simulink model "gmStateSpaceHDL_buckboost_convert_fixpt_vnl"  (R2025a)
settings: Solver=FixedStepDiscrete  StartTime=0.0  StopTime=0.005  FixedStep=Auto  RelTol=1e-3  AbsTol=1e-3
InitFcn:
  | load('C:\Users\bensa\Desktop\PI3_FPGA_BuckConverter\sschdl\buckboost_convert\stateSpaceParameters.mat');
values from neighbouring files (symbols this model uses):
  stateSpaceParameters_1 =     [stateSpaceParameters.mat]
libraries: fl_lib x5, hdlssclib x4, ee_lib x4, nesl_utility x4, simulink x3, hdlsllib x3
CloseFcn:
  | clear stateSpaceParameters_1
settings Model: MinMaxOverflowLogging=MinMaxAndOverflow  FPTRunName=EmbeddedRun1  Creator=bensa  LastModifiedBy=bensa
settings SolverCC: AutoScaleAbsTol=off  AlgebraicLoopSolver=TrustRegion  MaxZcPerStep=1.0
settings OptimizationCC: BlockReduction=off  ConditionallyExecuteInputs=off  DefaultParameterBehavior=Inlined  InheritOutputTypeSmallerThanSingle=on
settings DebuggingCC: SignalRangeChecking=warning  ArtificialAlgebraicLoopMsg=error  SingleTaskRateTransMsg=error  ParameterOverflowMsg=warning  ParameterUnderflowMsg=warning  UnconnectedInputMsg=warning  UnconnectedOutputMsg=warning  UnconnectedLineMsg=warning  SymbolicDimsDataTypeCodeGenerationDiagnostic=none
settings HardwareCC: ProdBitPerPointer=32.0  ProdBitPerSizeT=32.0  ProdBitPerPtrDiffT=32.0  ProdLargestAtomicFloat=None  ProdIntDivRoundTo=Undefined  ProdEndianess=Unspecified  ProdWordSize=32.0  ProdHWDeviceType=ASIC/FPGA->ASIC/FPGA  TargetBitPerPointer=64.0  TargetBitPerSizeT=64.0  TargetBitPerPtrDiffT=64.0  TargetLongLongMode=on  TargetIntDivRoundTo=Zero  TargetEndianess=LittleEndian  TargetWordSize=64.0  TargetHWDeviceType=Custom Processor->MATLAB Host Computer  ProdEqTarget=off
settings ModelReferenceCC: EnableRefExpFcnMdlSchedulingChecks=on
settings SFSimCC: CustomCodeUndefinedFunction=UseInterfaceOnly
settings RTWCC: GPUComputeCapability=3.5  DLArmComputeVersion=19.05
settings SimscapeCC: SimscapeLogType=all  SimscapeLogSimulationStatistics=on  SimscapeLogDataHistory=10000.0

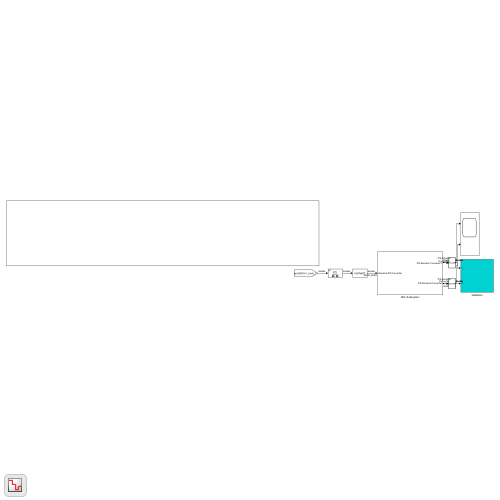
[thumbnail: Simulink's stored preview of the top-level diagram]
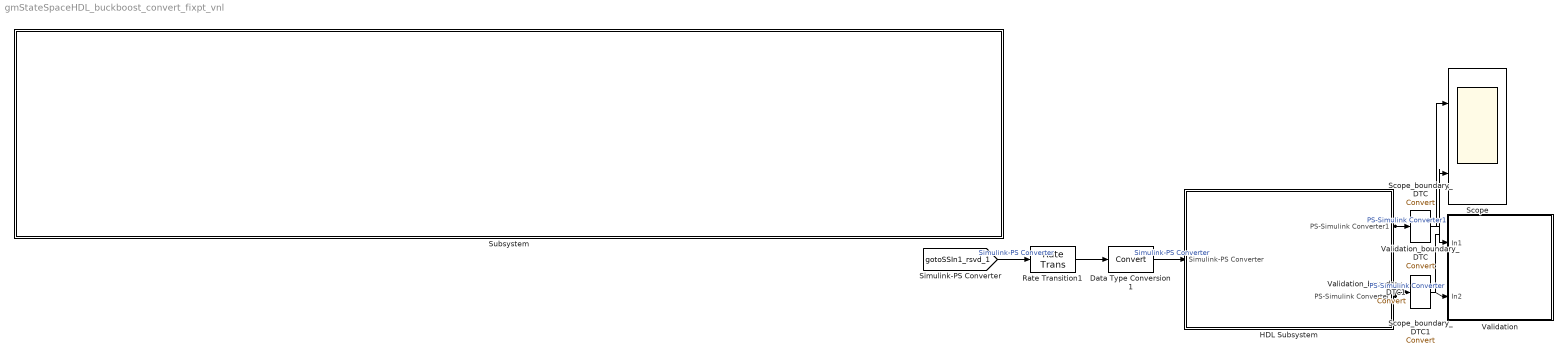
== system gmStateSpaceHDL_buckboost_convert_fixpt_vnl ==
  Data Type Conversion1 : DataTypeConversion  RndMeth=Nearest  SaturateOnIntegerOverflow=off
  HDL Subsystem : Subsystem  DataTypeOverride=Off  MinMaxOverflowLogging=MinMaxAndOverflow
  Rate Transition1 : RateTransition  OutPortSampleTime=5e-08
  Scope : Scope  NumInputPorts=2
      settings: DataLoggingVariableName=ScopeData2  DataLoggingSaveFormat=Array
  Scope_boundary_DTC : DataTypeConversion
  Scope_boundary_DTC1 : DataTypeConversion
  Subsystem : Subsystem
  Validation : Subsystem
  Validation_boundary_DTC : DataTypeConversion
  Validation_boundary_DTC1 : DataTypeConversion
  wires:
  HDL Subsystem/2(PS-Simulink Converter) -> Scope_boundary_DTC1/1, Validation_boundary_DTC1/1  "PS-Simulink Converter"
  Data Type Conversion1/1 -> HDL Subsystem/1(Simulink-PS Converter)  "Simulink-PS Converter"
  [gotoSSIn1_rsvd_1] -> Rate Transition1/1  "Simulink-PS Converter"
  Rate Transition1/1 -> Data Type Conversion1/1
  HDL Subsystem/1(PS-Simulink Converter1) -> Scope_boundary_DTC/1, Validation_boundary_DTC/1  "PS-Simulink Converter1"
  Scope_boundary_DTC/1 -> Scope/1
  Validation_boundary_DTC/1 -> Validation/1(In1)
  Scope_boundary_DTC1/1 -> Scope/2
  Validation_boundary_DTC1/1 -> Validation/2(In2)

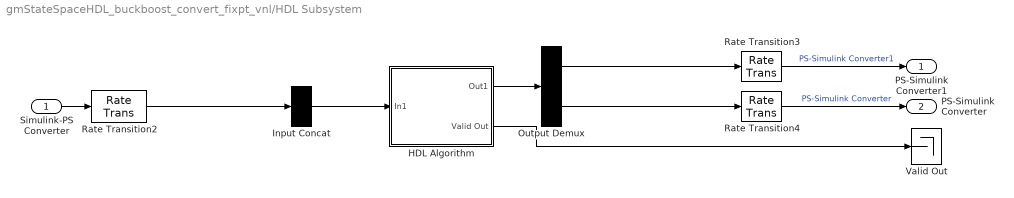
== system gmStateSpaceHDL_buckboost_convert_fixpt_vnl/HDL Subsystem ==
  Simulink-PS Converter : Inport  OutDataTypeStr=fixdt(0,32,29)
  HDL Algorithm : Subsystem
  Input Concat : Concatenate  NumInputs=1
  Output Demux : Demux  Outputs=2
  Rate Transition2 : RateTransition  Integrity=off  OutPortSampleTimeOpt=Multiple of input port sample time  OutPortSampleTimeMultiple=1/2
  Rate Transition3 : RateTransition  OutPortSampleTimeOpt=Multiple of input port sample time  OutPortSampleTimeMultiple=2
  Rate Transition4 : RateTransition  OutPortSampleTimeOpt=Multiple of input port sample time  OutPortSampleTimeMultiple=2
  Valid Out : Terminator
  PS-Simulink Converter1 : Outport
  PS-Simulink Converter : Outport  Port=2
  wires:
  Rate Transition3/1 -> PS-Simulink Converter1/1  "PS-Simulink Converter1"
  HDL Algorithm/1(Out1) -> Output Demux/1
  Input Concat/1 -> HDL Algorithm/1(In1)
  HDL Algorithm/2(Valid Out) -> Valid Out/1
  Rate Transition2/1 -> Input Concat/1
  Simulink-PS Converter/1 -> Rate Transition2/1
  Output Demux/2 -> Rate Transition4/1
  Output Demux/1 -> Rate Transition3/1
  Rate Transition4/1 -> PS-Simulink Converter/1  "PS-Simulink Converter"

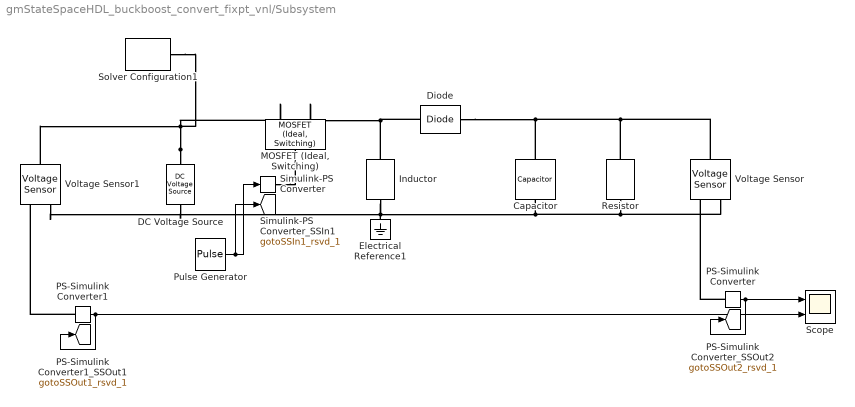
== system gmStateSpaceHDL_buckboost_convert_fixpt_vnl/Subsystem ==
  Capacitor : fl_lib/Electrical/Electrical Elements/Capacitor  c=47 uF  r=1e-6 Ohm  g=0 1/Ohm  i_specify=off  i_priority=None  i=0 A  i_nominal_specify=off  i_nominal_value=1  i_nominal_unit=A  v_specify=off  v_priority=None  v=0 V  v_nominal_specify=off  v_nominal_value=1  v_nominal_unit=V  vc_specify=off  vc_priority=High  vc=0 V  vc_nominal_specify=off  vc_nominal_value=1  vc_nominal_unit=V
  DC Voltage Source : ee_lib/Additional Components/SPICE Sources/DC Voltage Source  DC=5 V
  Diode : ee_lib/Semiconductors & Converters/Diode  ModelType=ee.enum.diode.modelType.pwl  TableType=ee.enum.diode.tableType.IfMat  IfMat=[.07, .12, .19, 1.75, 4.24, 7.32, 11.2; .16, .3, .72, 2.14, 5.02, 8.35, 13.12] A  VfMat=[.9, 1.15, 1.25, 1.5, 1.75, 2.17, 2.6, 2.85; .58, .68, .75, 1.1, 1.38, 1.77, 2.27, 2.7] V  TjVec=[25, 125] degC  VfVec=[.5, .7, .9, 1.3, 1.7, 2.1, 2.5] V  IfVec=[.1, .2, .5, 1, 2, 4, 7, 10] A  IrMat=[1e-06, 2e-06, 5e-06, 1e-05, 2.5e-05, 5e-05, .0001; 2e-06, 5e-06, 1e-05, 4e-05, 8e-05, .0002, .0005] A  VrMat=[10, 100, 200, 250, 300, 325, 350; 10, 70, 160, 220, 270, 300, 320] V  VrVec=[10, 20, 40, 50, 70, 80, 100] V  IrVec=[1e-06, 2e-06, 5e-06, 1e-05, 2e-05, 5e-05, .0001] A  Vf=0.7 V  Ron=0.1 Ohm  Goff=1e-8 S  prmExp=ee.enum.diode.expParam.useTwo  I12=[.0137, .545] A  V12=[.6, .7] V  RS=0 Ohm  Tmeas=298.15 K  IS=1e-12 A  ec=1  I1=0.0137 A  V1=0.6 V  N_series=1  N_parallel=1  ZenerEnable=false  Rz=0.3 Ohm  BV=inf V  C_param=ee.enum.diode.capParam.fixed  CJ=0 pF  CJ0=5 pF  Vvec=[.1, 10, 100] V  Cvec=[3.5, 1, .4] pF  VJ=1 V  Mgrad=0.5  FC=0.5  Q_param=ee.enum.diode.recoveryParam.off  iRM=-7.15 A  iF=4 A  didt=-750 A/us  trr_factor=3  trr=115 ns  Qrr=150 nA*s  Vr=-600 V  Ls=150 nH  Erec=0.03 J  TT=50 ns  tau=100 ns  T_param=ee.enum.diode.temperatureParam.off  Tdevice=298.15 K  I1_T2=0.245 A  V1_T2=0.5 V  IS_T2=1.25e-7 A  Tmeas2=125 degC  XTI_param=ee.enum.diode.xtiParam.pn  XTI=3  EG_param=ee.enum.diode.egapParam.material_si  EG=1.11 eV  dBVdT=0 V/K  enable_fault_input=simscape.enum.onoff.off  i_specify=off  i_priority=None  i=0 A  i_nominal_specify=off  i_nominal_value=1  i_nominal_unit=A  v_specify=off  v_priority=None  v=0 V  v_nominal_specify=off  v_nominal_value=1  v_nominal_unit=V  v_capacitor_specify=off  v_capacitor_priority=None  v_capacitor=0 V  v_capacitor_nominal_specify=off  v_capacitor_nominal_value=1  v_capacitor_nominal_unit=V  Qj_specify=off  Qj_priority=High  Qj=0 C  Qj_nominal_specify=off  Qj_nominal_value=1  Qj_nominal_unit=C  i_diode_specify=off  i_diode_priority=None  i_diode=0 A  i_diode_nominal_specify=off  i_diode_nominal_value=1  i_diode_nominal_unit=A  v_diode_specify=off  v_diode_priority=None  v_diode=0 V  v_diode_nominal_specify=off  v_diode_nominal_value=1  v_diode_nominal_unit=V  i_capacitor_specify=off  i_capacitor_priority=None  i_capacitor=0 A  i_capacitor_nominal_specify=off  i_capacitor_nominal_value=1  i_capacitor_nominal_unit=A  power_dissipated_specify=off  power_dissipated_priority=None  power_dissipated=0 W  power_dissipated_nominal_specify=off  power_dissipated_nominal_value=1  power_dissipated_nominal_unit=W  fidelity_level=ee.enum.diode.fidelity.includeChargeDyn  rec_loss_model=ee.enum.diode.reverseRecoveryModel.fixed  ErecVal=0 J  scaleWithIandV=true  ErecMat=zeros(2, 3) J  TjrecVec=[298.15, 398.15] K  IfrecVec=[.1, 1, 10] A  IrecVal=10 A  VrecVal=10 V  tFilter=1 / 1000 / 100 s  thermal_network_parameterization=ee.enum.thermalNetworkTopology.junctionCase  Rth=[0, 10] K/W  Rth_Cauer=[1, 3, 10] K/W  Rth_Foster=[.08, .14, .22, .16] K/W  thermal_mass_parameterization=ee.enum.thermalNetwork.timeconstant  thermal_mass=[0, 1] J/K  thermal_mass_Cauer=[.1, .3, 1] J/K  thermal_mass_Foster=[.001, .005, .05, .5] J/K  thermal_time_constant=[0, 10] s  thermal_time_constant_Cauer=[1, 3, 10] s  thermal_time_constant_Foster=[7e-05, .0007, .01, .08] s  thermal_mass_initial_temperatures=[25, 25] degC  thermal_mass_initial_temperatures_Cauer=[25, 25, 25] degC  junction_thermal_mass=0.01 J/K  Tvec_initial_Foster=[25, 25, 25, 25] degC  no_thermal_network=0  junction_temperature_specify=off  junction_temperature_priority=None  junction_temperature=25 degC  junction_temperature_nominal_specify=off  junction_temperature_nominal_value=1  junction_temperature_nominal_unit=degC
  Electrical Reference1 : fl_lib/Electrical/Electrical Elements/Electrical Reference
  Inductor : ee_lib/Passive/Inductor  l=100 uH  enable_L_tol=ee.enum.toleranceApplication.none  L_tol=20  tol_distribution=ee.enum.toleranceDistribution.uniform  nSigma=4  r=0 Ohm  g=1e-9 1/Ohm  enable_operating_limits=ee.enum.enable.no  operating_limit_action=ee.enum.passive.reportOpLim.warn  max_working_current=1 A  power_rating=1 W  i_L_specify=off  i_L_priority=High  i_L=0 A  i_L_nominal_specify=off  i_L_nominal_value=1  i_L_nominal_unit=A
  "MOSFET (Ideal, Switching)" : ee_lib/Semiconductors & Converters/MOSFET (Ideal, Switching)  port_option=ee.enum.controlport.ps  Rds=0.01 Ohm  Goff=1e-6 1/Ohm  Vth=2 V  diode_param=ee.enum.semiconductors.protectionDiode.external  diode_Vf=0.8 V  diode_Ron=0.001 Ohm  diode_Goff=1e-5 1/Ohm  diode_C=50e-9 F  diode_iRM=-235 A  diode_iF=300 A  diode_idot=-50 A/us  diode_trr_param=ee.enum.converters.diodeReverseParam.trr_factor  diode_trr_factor=3  diode_trr=15 us  diode_Qrr=1500 s*uA  ids_specify=off  ids_priority=None  ids=0 A  ids_nominal_specify=off  ids_nominal_value=1  ids_nominal_unit=A  vds_specify=off  vds_priority=None  vds=0 V  vds_nominal_specify=off  vds_nominal_value=1  vds_nominal_unit=V  vgs_specify=off  vgs_priority=None  vgs=0 V  vgs_nominal_specify=off  vgs_nominal_value=1  vgs_nominal_unit=V  thermal_loss_option=ee.enum.converters.thermalLossOption.constantvalues  Von_data=[0, 1.8, 3.2, 6, 10, 16; 0, 2, 5.5, 9.5, 15, 25] V  Tj=[298.15, 448.15] K  Iout_data=[0, 20, 40, 60, 80, 100] A  Eon_data=[0, 55.04, 124.57, 235.53, 362.12; 0, 71.25, 161.25, 304.88, 468.75] * 1e-6 J  Eoff_data=[0, 18, 30, 56.1, 76.5; 0, 22.5, 37.5, 70.13, 95.63] * 1e-6 J  Eon_data_3D=[zeros(2, 5, 3)] J  Eoff_data_3D=[zeros(2, 5, 3)] J  Tj_loss=[298.15, 448.15] K  Iout_data_loss=[0, 10, 20, 30, 40] A  tabulateWithVds=false  Vds_loss=[0, 150, 300] V  Eon_scalar=22.86e-3 J  Eoff_scalar=17.14e-3 J  Voff=300 V  Iout_scalar=600 A  useCurrentFromPreviousCycle=false  useVoltageFromPreviousCycle=false  diodeModelType=ee.enum.converters.diodeModelType.pwl  diodeTableType=ee.enum.diode.tableType.IfMat  diode_ReverseIVType=ee.enum.diode.diodeReverseIV.constant  diode_IfMat=[.07, .12, .19, 1.75, 4.24, 7.32, 11.2; .16, .3, .72, 2.14, 4.02, 6.35, 9.12] A  diode_VfMat=[.9, 1.15, 1.25, 1.5, 1.75, 2.17, 2.6, 2.85; .58, .68, .75, 1.1, 1.38, 1.77, 2.27, 2.7] V  diode_TjVec=[25, 125] degC  diode_VfVec=[.5, .7, .9, 1.3, 1.7, 2.1, 2.5] V  diode_IfVec=[.1, .2, .5, 1, 2, 4, 7, 10] A  diode_IrMat=[1e-06, 2e-06, 5e-06, 1e-05, 2.5e-05, 5e-05, .0001; 2e-06, 5e-06, 1e-05, 4e-05, 8e-05, .0002, .0005] A  diode_VrMat=[10, 100, 200, 250, 300, 325, 350; 10, 70, 160, 220, 270, 300, 320] V  diode_VrVec=[10, 20, 40, 50, 70, 80, 100] V  diode_IrVec=[1e-06, 2e-06, 5e-06, 1e-05, 2e-05, 5e-05, .0001] A  diode_Vr=-600 V  diode_Ls=150 nH  diode_Erec=0.03 J  diode_rec_loss_model=ee.enum.diode.reverseRecoveryModel.fixed  diode_ErecVal=0 J  diode_scaleWithIandV=true  diode_ErecMat=zeros(2, 3) J  diode_TjrecVec=[298.15, 398.15] K  diode_IfrecVec=[.1, 1, 10] A  diode_IrecVal=10 A  diode_VrecVal=10 V  diode_tFilter=1 / 1000 / 100 s  separateThermalPortForDiode=false  thermal_network_parameterization=ee.enum.thermalNetworkTopology.external  Rth=[.03, .2] K/W  Rth_Cauer=[.03, .1, .2] K/W  Rth_Foster=[.08, .14, .22, .16] K/W  thermal_mass_parameterization=ee.enum.thermalNetwork.timeconstant  thermal_mass=[3, 25] J/K  thermal_mass_Cauer=[3, 10, 25] J/K  thermal_mass_Foster=[.001, .005, .05, .5] J/K  thermal_time_constant=[.1, 5] s  thermal_time_constant_Cauer=[.1, 1, 5] s  thermal_time_constant_Foster=[7e-05, .0007, .01, .08] s  thermal_mass_initial_temperatures=[25, 25] degC  thermal_mass_initial_temperatures_Cauer=[25, 25, 25] degC  junction_thermal_mass=0.1 J/K  Tvec_initial_Foster=[25, 25, 25, 25] degC  RthDiode=[.03, .2] K/W  RthCauerDiode=[.03, .1, .2] K/W  RthFosterDiode=[.03, .2] K/W  thermalMassDiode=[3, 25] J/K  thermalMassCauerDiode=[3, 10, 25] J/K  thermalMassFosterDiode=[33, 50] J/K  thermalTauDiode=[.1, 5] s  thermalTauCauerDiode=[.1, 1, 5] s  thermalTauFosterDiode=[1, 10] s  thermalMassInitTempDiode=[25, 25] degC  thermalMassInitTempCauerDiode=[25, 25, 25] degC  junctionthermalMassDiode=0.1 J/K  TVecInitialFosterDiode=[25, 25, 25, 25] degC  no_thermal_network=0  mosfet_junction_temperature_specify=off  mosfet_junction_temperature_priority=None  mosfet_junction_temperature=25 degC  mosfet_junction_temperature_nominal_specify=off  mosfet_junction_temperature_nominal_value=1  mosfet_junction_temperature_nominal_unit=degC  diode_junction_temperature_specify=off  diode_junction_temperature_priority=None  diode_junction_temperature=25 degC  diode_junction_temperature_nominal_specify=off  diode_junction_temperature_nominal_value=1  diode_junction_temperature_nominal_unit=degC  Qj_specify=off  Qj_priority=None  Qj=0 W  Qj_nominal_specify=off  Qj_nominal_value=1  Qj_nominal_unit=W  accumulatedSwitchingLosses_specify=off  accumulatedSwitchingLosses_priority=None  accumulatedSwitchingLosses=0 J
  PS-Simulink Converter : nesl_utility/PS-Simulink Converter  PhysicalDomain=network_engine_domain  SubClassName=ps_output  LeftPortType=input  RightPortType=output  PseudoPeriodic=off  Frequencies=[]  VectorFormat=inherit  Unit=inherit  AffineConversion=off
  PS-Simulink Converter1 : nesl_utility/PS-Simulink Converter  PhysicalDomain=network_engine_domain  SubClassName=ps_output  LeftPortType=input  RightPortType=output  PseudoPeriodic=off  Frequencies=[]  VectorFormat=inherit  Unit=inherit  AffineConversion=off
  Pulse Generator : DiscretePulseGenerator  Amplitude=5  Period=200  PulseWidth=.40*200  SampleTime=50e-9
  Resistor : fl_lib/Electrical/Electrical Elements/Resistor  R=24 Ohm  i_specify=off  i_priority=None  i=0 A  i_nominal_specify=off  i_nominal_value=1  i_nominal_unit=A  v_specify=off  v_priority=None  v=0 V  v_nominal_specify=off  v_nominal_value=1  v_nominal_unit=V
  Scope : Scope  NumInputPorts=2
      settings: ActiveDisplayYMinimum=-5.8064728350082557  ActiveDisplayYMaximum=6.2007192038898058
  Simulink-PS Converter : nesl_utility/Simulink-PS Converter  PhysicalDomain=network_engine_domain  SubClassName=ps_input  LeftPortType=input  RightPortType=output  PseudoPeriodic=off  Frequencies=[]  NoiseDistribution=none  NoiseParameters=[]  Unit=1  AffineConversion=off  FilteringAndDerivatives=provide  SimscapeFilterOrder=1  InputFilterTimeConstant=0.001  UdotUserProvided=0
  Solver Configuration1 : nesl_utility/Solver Configuration  PhysicalDomain=network_engine_domain  SubClassName=solver  LeftPortType=input  RightPortType=generic  Tones=[]  Harmonics=[]  SimulateNoise=off  Profile=off  UseLocalSampling=off  EnableSwitchedLinearOptims=on  FrequencyDomain=off  UseCCode=off  RelTol=0.001  AbsTol=0.001  MinStep=1e-09  ToWorkspace=off  RevertToSquareIcSolve=off  NumHomotopyIterations=100  PhasorMode=off  PhasorModeNumHarmonics=1  ConsistencySolver=NEWTON_XTOL_AFTER_FTOL  IndexReductionMethod=DerivativeReplacement  DoDC=off  ResidualTolerance=1e-09  ConsistencyTolSource=GLOBAL  ConsistencyAbsTol=0.001  ConsistencyRelTol=0.001  ConsistencyTolFactor=0.001  UseLocalSolver=on  LocalSolverChoice=NE_BACKWARD_EULER_ADVANCER  ResolveIndetEquations=on  FunctionEvalNumThread=1  LocalSolverSampleTime=50e-9  DoFixedCost=on  MaxNonlinIter=2  MaxModeIter=2  ComputeImpulses=off  ImpulseIterations=2  LinearAlgebra=auto  LinearAlgebraNumThread=0  EquationFormulation=NE_TIME_EF  DelaysMemoryBudget=1024  AutomaticFiltering=on  FilteringTimeConstant=0.001  PartitionStorageMethod=AS_NEEDED  PartitionMemoryBudget=1024  PartitionMethod=ROBUST  MultibodyUseLocalSolver=off  MultibodyLocalSolverChoice=ODE1  MultibodyLocalSolverSampleTime=0.001
  Voltage Sensor : fl_lib/Electrical/Electrical Sensors/Voltage Sensor
  Voltage Sensor1 : fl_lib/Electrical/Electrical Sensors/Voltage Sensor
  tag scope: gotoSSIn1_rsvd_1=global, gotoSSOut1_rsvd_1=global, gotoSSOut2_rsvd_1=global
  wires:
  Pulse Generator/1 -> Simulink-PS Converter/1, [gotoSSIn1_rsvd_1]
  PS-Simulink Converter1/1 -> Scope/2, [gotoSSOut1_rsvd_1]
  PS-Simulink Converter/1 -> Scope/1, [gotoSSOut2_rsvd_1]
  connections:
  Voltage Sensor/LConn1 -- Capacitor/LConn1 -- Diode/LConn1 -- Resistor/LConn1
  Voltage Sensor/RConn2 -- Capacitor/RConn1 -- Electrical Reference1/LConn1 -- Inductor/RConn1 -- Voltage Sensor1/RConn2 -- DC Voltage Source/RConn1 -- Resistor/RConn1
  PS-Simulink Converter/LConn1 -- Voltage Sensor/RConn1
  DC Voltage Source/LConn1 -- "MOSFET (Ideal, Switching)"/RConn1 -- Solver Configuration1/RConn1 -- Voltage Sensor1/LConn1
  PS-Simulink Converter1/LConn1 -- Voltage Sensor1/RConn1
  Inductor/LConn1 -- "MOSFET (Ideal, Switching)"/RConn2 -- Diode/RConn1
  Simulink-PS Converter/RConn1 -- "MOSFET (Ideal, Switching)"/LConn1

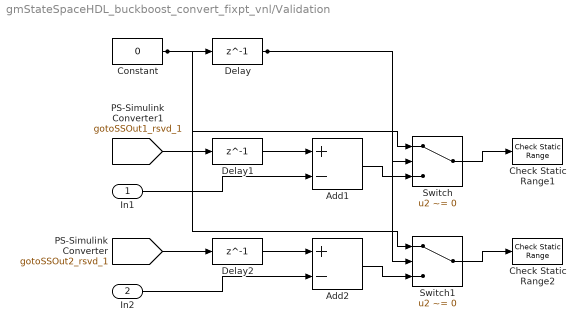
== system gmStateSpaceHDL_buckboost_convert_fixpt_vnl/Validation ==
  In1 : Inport
  In2 : Inport  Port=2
  Add1 : Sum  Inputs=+-
  Add2 : Sum  Inputs=+-
  Check Static Range1 : simulink/Model Verification/Check  Static Range  Description=-0.001 <= u <= 0.001  max=0.001  max_included=on  min=-0.001  min_included=on  enabled=on  stopWhenAssertionFail=off  export=off  icon=graphic
      settings: LibrarySourceBlock=|
      | hdlsllib/Model
      | Verification/Check
      | Static Range
  Check Static Range2 : simulink/Model Verification/Check  Static Range  Description=-0.001 <= u <= 0.001  max=0.001  max_included=on  min=-0.001  min_included=on  enabled=on  stopWhenAssertionFail=off  export=off  icon=graphic
      settings: LibrarySourceBlock=|
      | hdlsllib/Model
      | Verification/Check
      | Static Range
  Constant : Constant  Value=0  SampleTime=5e-08
  Delay : Delay  DelayLength=1  InitialCondition=1
  Delay1 : Delay  DelayLength=1
  Delay2 : Delay  DelayLength=1
  Switch : Switch  Criteria=u2 ~= 0  SaturateOnIntegerOverflow=off  InputSameDT=off
  Switch1 : Switch  Criteria=u2 ~= 0  SaturateOnIntegerOverflow=off  InputSameDT=off
  wires:
  Constant/1 -> Delay/1, Switch/1, Switch1/1
  [gotoSSOut1_rsvd_1] -> Delay1/1
  Delay1/1 -> Add1/1
  In1/1 -> Add1/2
  Add1/1 -> Switch/3
  Delay/1 -> Switch/2, Switch1/2
  Switch/1 -> Check Static Range1/1
  [gotoSSOut2_rsvd_1] -> Delay2/1
  Delay2/1 -> Add2/1
  In2/1 -> Add2/2
  Add2/1 -> Switch1/3
  Switch1/1 -> Check Static Range2/1

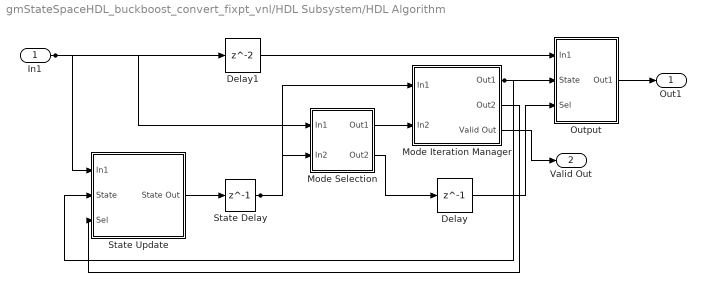
== system gmStateSpaceHDL_buckboost_convert_fixpt_vnl/HDL Subsystem/HDL Algorithm ==
  In1 : Inport  OutDataTypeStr=fixdt(0,32,29)
  Delay : Delay  DelayLength=1
  Delay1 : Delay
  Mode Iteration Manager : Subsystem
  Mode Selection : Subsystem
  Output : Subsystem
  State Delay : Delay  DelayLength=1  InitialCondition=single(stateSpaceParameters_1.X0)
  State Update : Subsystem
  Out1 : Outport  VectorParamsAs1DForOutWhenUnconnected=off
  Valid Out : Outport  Port=2  VectorParamsAs1DForOutWhenUnconnected=off
  wires:
  State Delay/1 -> Mode Iteration Manager/1(In1), Mode Selection/2(In2)
  Delay1/1 -> Output/1(In1)
  State Update/1(State Out) -> State Delay/1
  In1/1 -> Mode Selection/1(In1), Delay1/1, State Update/1(In1)
  Mode Selection/1(Out1) -> Mode Iteration Manager/2(In2)
  Mode Iteration Manager/2(Out2) -> State Update/3(Sel)
  Mode Iteration Manager/1(Out1) -> State Update/2(State), Output/2(State)
  Mode Selection/2(Out2) -> Delay/1
  Mode Iteration Manager/3(Valid Out) -> Valid Out/1
  Output/1(Out1) -> Out1/1
  Delay/1 -> Output/3(Sel)

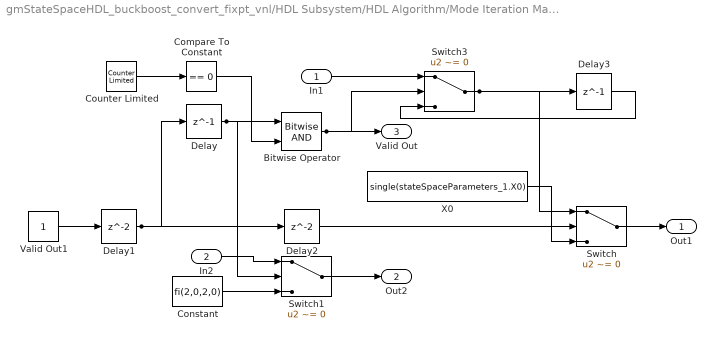
== system gmStateSpaceHDL_buckboost_convert_fixpt_vnl/HDL Subsystem/HDL Algorithm/Mode Iteration Manager ==
  In1 : Inport  LockScale=on
  In2 : Inport  Port=2  OutDataTypeStr=fixdt(0,2,0)  LockScale=on
  Bitwise Operator : simulink/Logic and Bit Operations/Bitwise Operator  logicop=AND  UseBitMask=off  NumInputPorts=2  BitMask=bin2dec('11011001')  BitMaskRealWorld=Stored Integer
      settings: LibrarySourceBlock=|
      | hdlsllib/Logic and Bit
      | Operations/Bitwise
      | Operator
  Compare To Constant : hdlsllib/Logic and Bit Operations/Compare To Constant  relop===  const=0  OutDataTypeStr=boolean
  Constant : Constant  Value=fi(2,0,2,0)  SampleTime=2.5e-08  LockScale=on
  Counter Limited : hdlsllib/Sources/Counter Limited  uplimit=1  tsamp=-1
  Delay : Delay  DelayLength=1
  Delay1 : Delay
  Delay2 : Delay
  Delay3 : Delay  DelayLength=1
  Switch : Switch  Criteria=u2 ~= 0  OutDataTypeStr=fixdt(1,32,25)  SaturateOnIntegerOverflow=off  InputSameDT=off
  Switch1 : Switch  Criteria=u2 ~= 0  SaturateOnIntegerOverflow=off  InputSameDT=off  OutDataTypeStr=Inherit: Same as first input
      settings: LockScale=on
  Switch3 : Switch  Criteria=u2 ~= 0  OutDataTypeStr=fixdt(1,32,28)  SaturateOnIntegerOverflow=off  InputSameDT=off
  Valid Out1 : Constant  OutDataTypeStr=boolean  SampleTime=2.5e-08
  X0 : Constant  Value=single(stateSpaceParameters_1.X0)  OutDataTypeStr=fixdt(0,32,29)  SampleTime=2.5e-08
  Out1 : Outport  OutDataTypeStr=fixdt(1,32,25)  VectorParamsAs1DForOutWhenUnconnected=off
  Out2 : Outport  Port=2  VectorParamsAs1DForOutWhenUnconnected=off
  Valid Out : Outport  Port=3  VectorParamsAs1DForOutWhenUnconnected=off
  wires:
  Valid Out1/1 -> Delay1/1
  Counter Limited/1 -> Compare To Constant/1
  Delay1/1 -> Delay/1, Delay2/1
  Compare To Constant/1 -> Bitwise Operator/2
  Delay/1 -> Switch1/2, Bitwise Operator/1
  In2/1 -> Switch1/1
  Constant/1 -> Switch1/3
  In1/1 -> Switch3/1
  Bitwise Operator/1 -> Valid Out/1, Switch3/2
  Delay2/1 -> Switch/2
  Switch1/1 -> Out2/1
  Switch3/1 -> Delay3/1, Switch/1
  X0/1 -> Switch/3
  Delay3/1 -> Switch3/3
  Switch/1 -> Out1/1

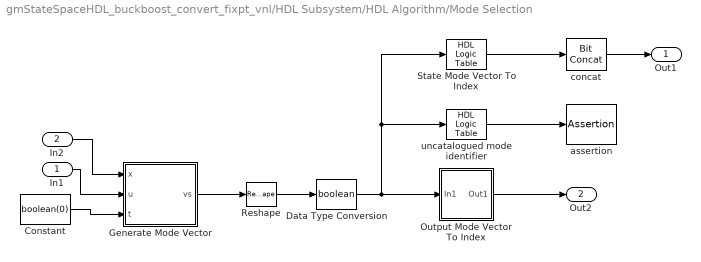
== system gmStateSpaceHDL_buckboost_convert_fixpt_vnl/HDL Subsystem/HDL Algorithm/Mode Selection ==
  In1 : Inport  OutDataTypeStr=fixdt(0,32,29)
  In2 : Inport  Port=2  LockScale=on
  Constant : Constant  Value=boolean(0)  SampleTime=2.5e-08
  Data Type Conversion : DataTypeConversion  OutDataTypeStr=boolean  RndMeth=Nearest  SaturateOnIntegerOverflow=off
  Generate Mode Vector : Subsystem  TreatAsAtomicUnit=on  Variant=on
  Output Mode Vector To Index : Subsystem
  Reshape : Reshape
  State Mode Vector To Index : hdlssclib/HDL Logic Table  InputTable=stateSpaceParameters_1.logicTableInput  OutputTable=stateSpaceParameters_1.logicTableOutput
  assertion : Assertion  StopWhenAssertionFail=off
  concat : hdlsllib/Logic and Bit Operations/Bit Concat  numInputs=1
  uncatalogued mode identifier : hdlssclib/HDL Logic Table  InputTable=stateSpaceParameters_1.logicTableInput  OutputTable=ones(size(stateSpaceParameters_1.logicTableOutput,1),1)
  Out1 : Outport  VectorParamsAs1DForOutWhenUnconnected=off  LockScale=on
  Out2 : Outport  Port=2  VectorParamsAs1DForOutWhenUnconnected=off
  wires:
  Data Type Conversion/1 -> State Mode Vector To Index/1, uncatalogued mode identifier/1, Output Mode Vector To Index/1(In1)
  State Mode Vector To Index/1 -> concat/1
  Reshape/1 -> Data Type Conversion/1
  uncatalogued mode identifier/1 -> assertion/1
  Output Mode Vector To Index/1(Out1) -> Out2/1
  concat/1 -> Out1/1
  In2/1 -> Generate Mode Vector/1(x)
  In1/1 -> Generate Mode Vector/2(u)
  Constant/1 -> Generate Mode Vector/3(t)
  Generate Mode Vector/1(vs) -> Reshape/1

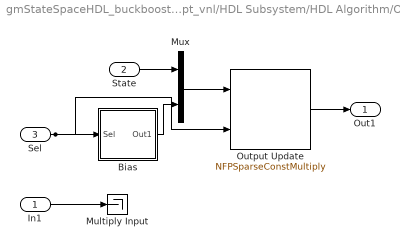
== system gmStateSpaceHDL_buckboost_convert_fixpt_vnl/HDL Subsystem/HDL Algorithm/Output ==
  In1 : Inport  OutDataTypeStr=fixdt(0,32,29)
  State : Inport  Port=2  OutDataTypeStr=fixdt(1,32,25)
  Sel : Inport  Port=3  LockScale=on
  Bias : Subsystem
  Multiply Input : Terminator
  Mux : Mux  Inputs=2
  Output Update : hdlssclib/NFPSparseConstMultiply  MatrixSource=Dialog  constMatrix=fi((([stateSpaceParameters_1.Cd repmat(eye(2),[1,1,1])])),0,32,31)  MatrixType=fixdt(0,32,31)  MatrixSize=[1 1]  ColumnIndices=[1]  RowIndices=[1]  PropDataType=fixdt(1,32,28)  defWL=32
  Out1 : Outport  VectorParamsAs1DForOutWhenUnconnected=off
  wires:
  Sel/1 -> Output Update/2, Bias/1(Sel)
  In1/1 -> Multiply Input/1
  State/1 -> Mux/1
  Bias/1(Out1) -> Mux/2
  Mux/1 -> Output Update/1
  Output Update/1 -> Out1/1

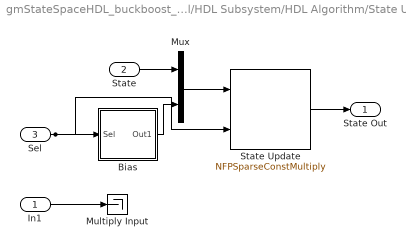
== system gmStateSpaceHDL_buckboost_convert_fixpt_vnl/HDL Subsystem/HDL Algorithm/State Update ==
  In1 : Inport  OutDataTypeStr=fixdt(0,32,29)
  State : Inport  Port=2  OutDataTypeStr=fixdt(1,32,25)
  Sel : Inport  Port=3  LockScale=on
  Bias : Subsystem
  Multiply Input : Terminator
  Mux : Mux  Inputs=2
  State Update : hdlssclib/NFPSparseConstMultiply  MatrixSource=Dialog  constMatrix=fi((([stateSpaceParameters_1.Ad repmat(eye(4),[1,1,4])])),1,32,20)  MatrixType=fixdt(1,32,20)  MatrixSize=[1 1]  ColumnIndices=[1]  RowIndices=[1]  PropDataType=fixdt(1,32,19)  defWL=32
  State Out : Outport  VectorParamsAs1DForOutWhenUnconnected=off
  wires:
  State/1 -> Mux/1
  Sel/1 -> State Update/2, Bias/1(Sel)
  In1/1 -> Multiply Input/1
  State Update/1 -> State Out/1
  Bias/1(Out1) -> Mux/2
  Mux/1 -> State Update/1

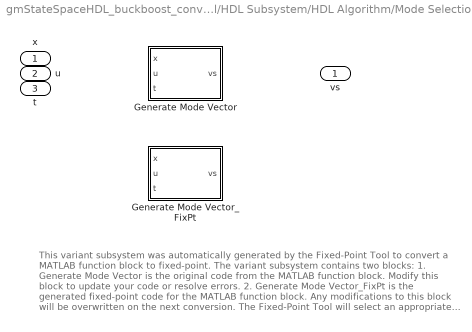
== system gmStateSpaceHDL_buckboost_convert_fixpt_vnl/HDL Subsystem/HDL Algorithm/Mode Selection/Generate Mode Vector ==
  note: This variant subsystem was automatically generated by the Fixed-Point Tool to convert a MATLAB function block to fixed-point.
      |
      | The variant subsystem contains two blocks:
      | 1. Generate Mode Vector is the original code from the MATLAB function block. Modify this block to update your code or resolve errors.
      |
      | 2. Generate Mode Vector_FixPt is the generated fixed-point code for the MATLAB function block. Any modifications to this block will be overwritten on the next conversion.
      |
      | The Fixed-Point Tool will select an appropriate variant based on the Model Settings. Learn more.
  x : Inport
  u : Inport  Port=2
  t : Inport  Port=3
  Generate Mode Vector : MATLAB Function  TreatAsAtomicUnit=on  VariantControl=false()
  Generate Mode Vector_FixPt : MATLAB Function  TreatAsAtomicUnit=on  VariantControl=(default)
  vs : Outport

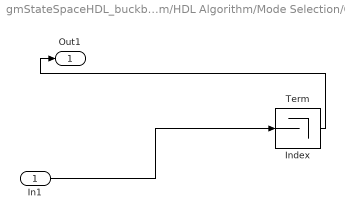
== system gmStateSpaceHDL_buckboost_convert_fixpt_vnl/HDL Subsystem/HDL Algorithm/Mode Selection/Output Mode Vector To Index ==
  In1 : Inport
  Index : Constant  Value=fi(0,0,1,0)  SampleTime=2.5e-08  LockScale=on
  Term : Terminator
  Out1 : Outport  VectorParamsAs1DForOutWhenUnconnected=off
  wires:
  In1/1 -> Term/1
  Index/1 -> Out1/1

== system gmStateSpaceHDL_buckboost_convert_fixpt_vnl/HDL Subsystem/HDL Algorithm/Output/Bias ==
  Sel : Inport  LockScale=on
  Bias : Constant  Value=single(stateSpaceParameters_1.Y0d)  OutDataTypeStr=fixdt(1,32,25)  SampleTime=2.5e-08
  Terminator : Terminator
  Out1 : Outport  VectorParamsAs1DForOutWhenUnconnected=off
  wires:
  Sel/1 -> Terminator/1
  Bias/1 -> Out1/1

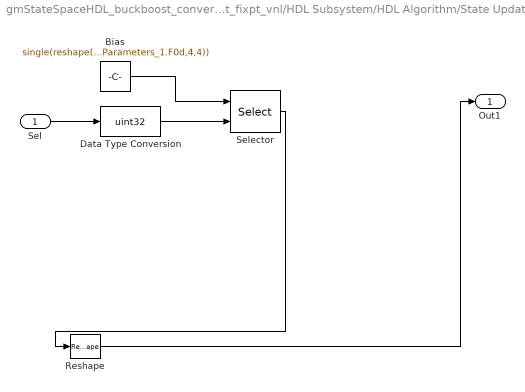
== system gmStateSpaceHDL_buckboost_convert_fixpt_vnl/HDL Subsystem/HDL Algorithm/State Update/Bias ==
  Sel : Inport  LockScale=on
  Bias : Constant  Value=single(reshape(stateSpaceParameters_1.F0d,4,4))  OutDataTypeStr=fixdt(1,32,25)  SampleTime=2.5e-08
  Data Type Conversion : DataTypeConversion  OutDataTypeStr=uint32  RndMeth=Nearest  SaturateOnIntegerOverflow=off
  Reshape : Reshape
  Selector : Selector  NumberOfDimensions=2  IndexMode=Zero-based  InputPortWidth=3  IndexOptions=Select all,Index vector (port)  Indices=[1 3]  OutputSizes=1
  Out1 : Outport  VectorParamsAs1DForOutWhenUnconnected=off
  wires:
  Selector/1 -> Reshape/1
  Bias/1 -> Selector/1
  Sel/1 -> Data Type Conversion/1
  Data Type Conversion/1 -> Selector/2
  Reshape/1 -> Out1/1

== matlab function gmStateSpaceHDL_buckboost_convert_fixpt_vnl/HDL Subsystem/HDL Algorithm/Mode Selection/Generate Mode Vector/Generate Mode Vector ==
  data: x input; u input; vs output; t input
function vs = compute_modes(x, u, t)

  tmp1 = (x(1) + ((1e-06) .* x(3)) + ((-1.0) .* x(4)));
  tmp2 = u(1);

  v1 = (tmp1 > (0.7));
  v2 = (tmp2 > (2.0));

  vs = [v1 v2];

end

== matlab function gmStateSpaceHDL_buckboost_convert_fixpt_vnl/HDL Subsystem/HDL Algorithm/Mode Selection/Generate Mode Vector/Generate Mode Vector_FixPt ==
  settings: fimath=fimath('RoundingMethod', 'Floor', 'OverflowAction', 'Wrap', 'ProductMode', 'FullPrecision', 'MaxProductWordLength', 128, 'SumMode', 'FullPrecision', 'MaxSumWordLength', 128)
  data: x input; u input; vs output; t input
%auto-generated
%#codegen
function vs = compute_modes_fixpt(x, u, t)

  fm = get_fimath();
  u = fi(u, 0, 32, 29, fm);

  tmp1 = (x(1) + ((fi(1e-06, 0, 16, 35, fm)) .* x(3)) + ((fi(-1.0, 1, 2, 0, fm)) .* x(4)));
  tmp2 = fi(u(1), 0, 32, 29, fm);

  v1 = (tmp1 > (fi(0.7, 0, 16, 16, fm)));
  v2 = (tmp2 > (fi(2.0, 0, 2, 0, fm)));

  vs = [v1 v2];

end


function fm = get_fimath()
	fm = fimath('RoundingMethod', 'Floor',...
	     'OverflowAction', 'Wrap',...
	     'ProductMode','FullPrecision',...
	     'MaxProductWordLength', 128,...
	     'SumMode','FullPrecision',...
	     'MaxSumWordLength', 128);
end
